simulink model "ELS_Testbench"  (R2021a)
settings: Solver=VariableStepAuto  StartTime=0.0  StopTime=10  FixedStep=Tsample  MaxStep=100e-4  RelTol=1e-3
values from neighbouring files (symbols this model uses):
  EncMaxSteps = 16777216    [ELS_Konstanten.m]
  EncOrTime = EncMaxSteps /(4096 * (RPM/60))    (= 144.564705882)    [ELS_Konstanten.m]
  TSampleRTM = 0.1e-3    (= 0.0001)    [ELS_Konstanten.m]
  TSampleStepper = 5e-6    (= 5e-06)    [ELS_Konstanten.m]
undefined symbols (not defined in the file or in its folder): sigbuilder_block
libraries: fl_lib x12, nesl_utility x5, simulink x2, ee_lib x2
settings Model: PacingRate=0.001800  OrderedModelArguments=off  Creator=lu  LastModifiedBy=lu
settings SolverCC: AlgebraicLoopSolver=TrustRegion  AutoInsertRateTranBlk=on
settings DebuggingCC: SFMachineParentedDataDiag=warning

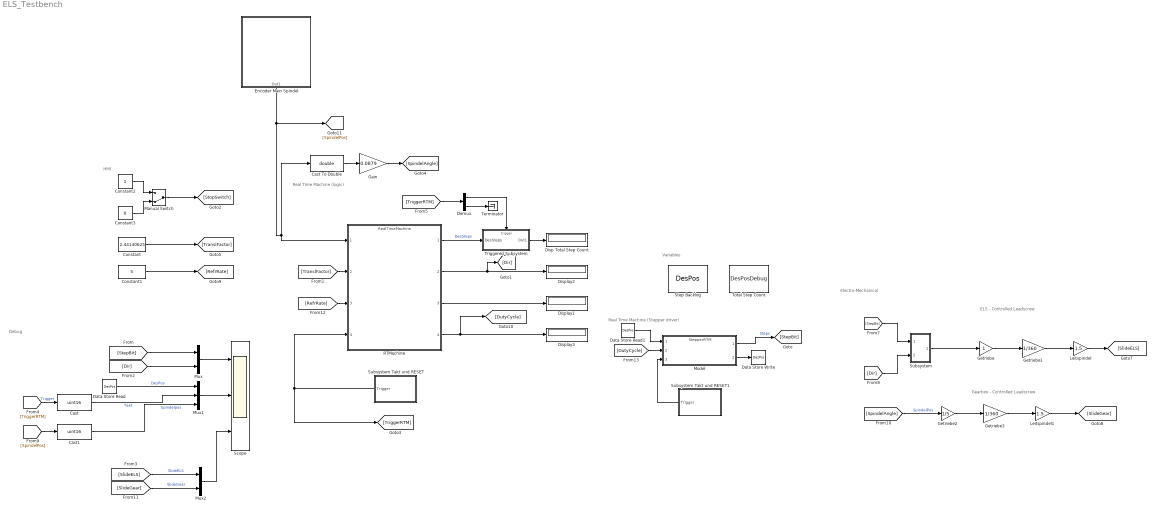
== system ELS_Testbench ==
  note: ELS - Controlled Leadscrew
  note: Electro-Mechanical
  note: Debug
  note: HMI
  note: Real Time Machine (Stepper driver)
  note: Real Time Machine (logic)
  note: Variables
  note: Gearbox - Controlled Leadscrew
  Cast : DataTypeConversion  OutDataTypeStr=uint16
  Cast To Double : DataTypeConversion  OutDataTypeStr=double
  Cast1 : DataTypeConversion  OutDataTypeStr=uint16
  Constant : Constant  Value=2.44140625  OutDataTypeStr=double
  Constant1 : Constant  Value=5  OutDataTypeStr=uint16
  Constant2 : Constant  OutDataTypeStr=boolean
  Constant3 : Constant  Value=0  OutDataTypeStr=boolean
  Data Store Read : DataStoreRead  DataStoreName=DesPos  IndexOptions=Index vector (dialog)  Indices=1  OutputSizes=1
  Data Store Read1 : DataStoreRead  DataStoreName=DesPos  IndexOptions=Index vector (dialog)  Indices=1  OutputSizes=1
  Data Store Write : DataStoreWrite  DataStoreName=DesPos  IndexOptions=Index vector (dialog)  Indices=1  OutputSizes=1
  Demux : Demux  Outputs=2
  Disp Total Step Count : Display
  Display1 : Display
  Display2 : Display
  Display3 : Display
  Encoder Main Spindel : Subsystem
  Gain : Gain  Gain=0.0879
  Getriebe : Gain
  Getriebe1 : Gain  Gain=1/360
  Getriebe2 : Gain  Gain=1/5
  Getriebe3 : Gain  Gain=1/360
  Leitspindel : Gain  Gain=1.5
  Leitspindel1 : Gain  Gain=1.5
  Manual Switch : ManualSwitch  CurrentSetting=0
  Model : ModelReference  ModelNameDialog=StepperRTM.slx  SimulationMode=Normal  ModelReferenceVersion=2.134
  Mux : Mux  Inputs=2
  Mux1 : Mux  Inputs=3
  Mux2 : Mux  Inputs=2
  RTMachine : ModelReference  ModelNameDialog=RealTimeMachine.slx  SimulationMode=Normal  ModelReferenceVersion=2.233
  Scope : Scope  NumInputPorts=3
  Step Backlog : DataStoreMemory  DataStoreName=DesPos  ReadBeforeWriteMsg=warning  WriteAfterWriteMsg=warning  WriteAfterReadMsg=warning  ShowAdditionalParam=off
  Subsystem : Subsystem
  Subsystem Takt und RESET : Subsystem
  Subsystem Takt und RESET1 : Subsystem
  Terminator : Terminator
  Total Step Count : DataStoreMemory  DataStoreName=DesPosDebug  ReadBeforeWriteMsg=warning  WriteAfterWriteMsg=warning  WriteAfterReadMsg=warning  ShowAdditionalParam=off
  Triggered Subsystem : Subsystem  TreatAsAtomicUnit=on
  wires:
  Constant3/1 -> Manual Switch/2
  Constant2/1 -> Manual Switch/1
  Subsystem Takt und RESET/1(Trigger) -> RTMachine/4, [TriggerRTM]
  Model/1 -> [StepBit]  "Steps"
  [StepBit] -> Mux/1
  Mux/1 -> Scope/1
  Subsystem Takt und RESET1/1(Trigger) -> Model/3
  [Dir] -> Mux/2
  RTMachine/1 -> Triggered Subsystem/1(DesSteps)  "DesSteps"
  [TriggerRTM] -> Demux/1
  Demux/1 -> Triggered Subsystem/Trigger
  Demux/2 -> Terminator/1
  Triggered Subsystem/1(Out1) -> Disp Total Step Count/1
  Encoder Main Spindel/1(Out1) -> [SpindelPos], Cast To Double/1, RTMachine/1
  [TranslFactor] -> RTMachine/2
  Manual Switch/1 -> [StopSwitch]
  Constant/1 -> [TranslFactor]
  [StepBit] -> Subsystem/1(In1)
  [Dir] -> Subsystem/2(In2)
  Subsystem/1(theta) -> Getriebe/1
  Gain/1 -> [SpindelAngle]
  Data Store Read/1 -> Mux1/1  "DesPos"
  Mux1/1 -> Scope/2
  Cast To Double/1 -> Gain/1
  Getriebe/1 -> Getriebe1/1
  Getriebe1/1 -> Leitspindel/1
  Mux2/1 -> Scope/3
  Leitspindel/1 -> [SlideELS]
  [SlideELS] -> Mux2/1  "SlideELS"
  Getriebe2/1 -> Getriebe3/1
  Getriebe3/1 -> Leitspindel1/1
  [SpindelAngle] -> Getriebe2/1  "SpindelPos"
  Leitspindel1/1 -> [SlideGear]
  [SlideGear] -> Mux2/2  "SlideGear"
  Constant1/1 -> [RefrRate]
  [DutyCycle] -> Model/2
  Model/2 -> Data Store Write/1
  Data Store Read1/1 -> Model/1
  [TriggerRTM] -> Cast/1  "Trigger"
  Cast/1 -> Mux1/2  "Takt"
  Cast1/1 -> Mux1/3  "Spindelpos"
  [SpindelPos] -> Cast1/1
  RTMachine/4 -> Display3/1, [DutyCycle]
  [RefrRate] -> RTMachine/3
  RTMachine/2 -> [Dir], Display2/1
  RTMachine/3 -> Display1/1

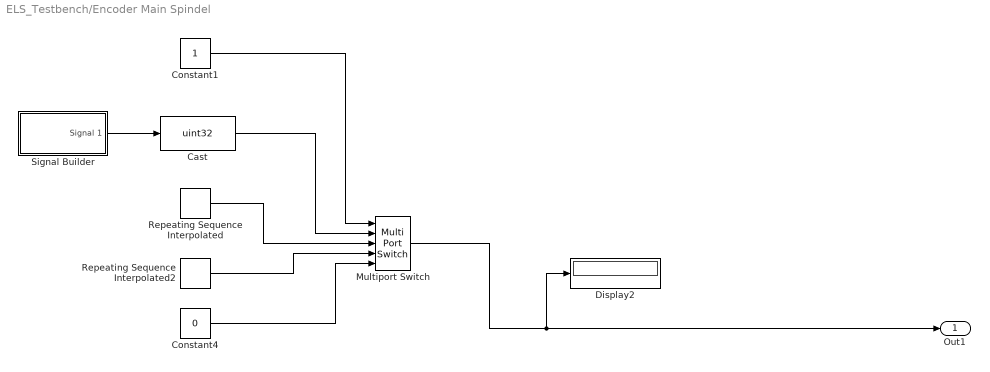
== system ELS_Testbench/Encoder Main Spindel ==
  Cast : DataTypeConversion  OutDataTypeStr=uint32
  Constant1 : Constant
  Constant4 : Constant  Value=0  OutDataTypeStr=uint32
  Display2 : Display
  Multiport Switch : MultiPortSwitch  Inputs=4
  Repeating Sequence Interpolated : simulink/Sources/Repeating Sequence Interpolated  OutValues=[0 EncMaxSteps/2 EncMaxSteps].'  TimeValues=[0 EncOrTime/2 EncOrTime].'  LookUpMeth=Interpolation-Use End Values  tsamp=TSampleRTM  OutMin=[]  OutMax=[]  OutDataTypeStr=uint32  OutputDataTypeScalingMode=uint32  OutDataType=fixdt(0,8)  OutScaling=2^-10
  Repeating Sequence Interpolated2 : simulink/Sources/Repeating Sequence Interpolated  OutValues=[EncMaxSteps EncMaxSteps/2 0].'  TimeValues=[0 EncOrTime/2 EncOrTime].'  LookUpMeth=Interpolation-Use End Values  tsamp=TSampleRTM  OutMin=[]  OutMax=[]  OutDataTypeStr=uint32  OutputDataTypeScalingMode=uint32  OutDataType=fixdt(0,8)  OutScaling=2^-10
  Signal Builder : Subsystem  Tag=STV Subsys  LoadFcn=sigbuilder_block('load');  StartFcn=sigbuilder_block('start');  StopFcn=sigbuilder_block('stop');  ClipboardFcn=sigbuilder_block('clipboard');  mask(Sigbuilder block){tuvar=[0:10]}
      mask help: Simulink:masks:SigbuilderBlock_MD
      mask init:
      | if ~strcmp(get_param(bdroot(gcbh),'SimulationStatus'),'stopped') tuvar = sigbuilder_block('maskInit'); end
      settings: CopyFcn=sigbuilder_block('copy');  DeleteFcn=sigbuilder_block('delete');  ModelCloseFcn=sigbuilder_block('modelClose');  PreSaveFcn=sigbuilder_block('preSave');  PauseFcn=sigbuilder_block('pause');  ContinueFcn=sigbuilder_block('continue');  NameChangeFcn=sigbuilder_block('namechange');  OpenFcn=sigbuilder_block('open',[437.6 199.2 550.4 400 ]);  CloseFcn=sigbuilder_block('close');
      mask Display: plot(0, 0, 100, 100,[2, 2, 32, 32, 2], [68, 8, 8, 68, 68],[32, 2], [38, 38], [32, 19, 2],[53, 60, 44], [32, 17, 17, 2],[16, 16, 31, 31]);txt = getActiveGroup(gcbh);text(2, 100, txt,'verticalAlignment', 'top');
  Out1 : Outport
  wires:
  Repeating Sequence Interpolated2/1 -> Multiport Switch/4
  Constant1/1 -> Multiport Switch/1
  Cast/1 -> Multiport Switch/2
  Constant4/1 -> Multiport Switch/5
  Multiport Switch/1 -> Out1/1, Display2/1
  Repeating Sequence Interpolated/1 -> Multiport Switch/3
  Signal Builder/1(Signal 1) -> Cast/1

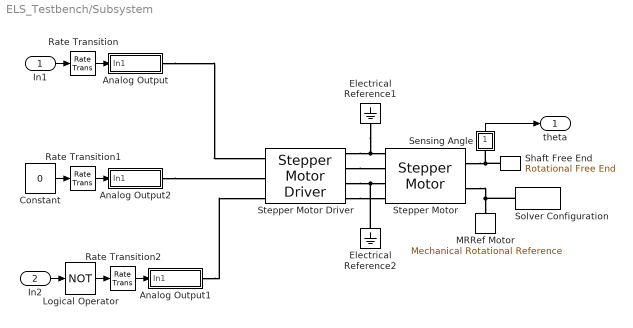
== system ELS_Testbench/Subsystem ==
  In1 : Inport
  In2 : Inport  Port=2
  Analog Output : Subsystem
  Analog Output1 : Subsystem
  Analog Output2 : Subsystem
  Constant : Constant  Value=0
  Electrical Reference1 : fl_lib/Electrical/Electrical Elements/Electrical Reference
  Electrical Reference2 : fl_lib/Electrical/Electrical Elements/Electrical Reference
  Logical Operator : Logic  Operator=NOT  AllPortsSameDT=off  OutDataTypeStr=boolean
  MRRef Motor : fl_lib/Mechanical/Rotational Elements/Mechanical Rotational Reference
  Rate Transition : RateTransition  Deterministic=off
  Rate Transition1 : RateTransition  Deterministic=off
  Rate Transition2 : RateTransition  Deterministic=off
  Sensing Angle : Subsystem
      mask Display: disp('a')
  Shaft Free End : fl_lib/Mechanical/Rotational Elements/Rotational Free End  w_specify=off  w_priority=None  w=0 rad/s  w_nominal_specify=off  w_nominal_unit=rad/s  w_nominal_value=1
      settings: SourceProductBaseCode=SS
  Solver Configuration : nesl_utility/Solver Configuration  PhysicalDomain=network_engine_domain  SubClassName=solver  LeftPortType=input  RightPortType=generic  Tones=[]  Harmonics=[]  SimulateNoise=off  Profile=off  UseLocalSampling=off  EnableSwitchedLinearOptims=on  FrequencyDomain=off  UseCCode=off  RelTol=0.001  AbsTol=1e-06  MinStep=1e-09  ToWorkspace=off  RevertToSquareIcSolve=off  NumHomotopyIterations=100  PhasorMode=off  PhasorModeNumHarmonics=1  DoDC=off  ResidualTolerance=1e-9  UseLocalSolver=off  LocalSolverChoice=NE_BACKWARD_EULER_ADVANCER  LocalSolverSampleTime=.001  DoFixedCost=off  MaxNonlinIter=3  MaxModeIter=2  ComputeImpulses=off  ImpulseIterations=2  LinearAlgebra=auto  EquationFormulation=NE_TIME_EF  DelaysMemoryBudget=1024  AutomaticFiltering=on  FilteringTimeConstant=3e-6  PartitionStorageMethod=AS_NEEDED  PartitionMemoryBudget=1024  PartitionMethod=FAST
      settings: SourceProductBaseCode=PW,SS
  Stepper Motor : ee_lib/Electromechanical/Reluctance & Stepper/Stepper Motor  Tag={'toolbox/physmod/elec/library/m/ee_lib_parts';'Electromechanical/Reluctance_and_Stepper/Stepper_Motor/Minebea/x08PM_K139BSTDCN.xml'}  step_or_av=1  w_vec=[0 1000 3000] rpm  T_vec=[2 2 1] N*m  assert_if_slipping=0  J_total=0.0001 kg*m^2  max_step_rate=10 Hz  Ra=6.5 Ohm  La=3.2 mH  Km=51.63 mN*m/A  Td=2.5 mN*m  Rm=Inf Ohm  Step=0.18 deg  J=2.9e-07 kg*m^2  B=2.65e-05 N*m/(rad/s)  speed0=0 rpm  theta0=0 deg  alpha=[0.00393 0.00393] 1/K  Tmeas=25 degC  T_vec2=[1.7 1.7 0.85] N*m  Tmeas2=125 degC  half_stepping=0  thermal_masses=[100 100] J/K  initial_temperatures=[25 25] degC  rotor_thermal_mass=50 J/K  rotor_initial_temperature=25 degC  Rm_percent_rotor=90
      settings: AttributesFormatString=Minebea:08PM-K139BSTDCN  SourceProductBaseCode=PS  InternalSimscapePortConfiguration="{\"Bottom\":[],\"Left\":[{\"id\":\"pA\",\"label\":\"A+\",\"type\":\"foundation.electrical.electrical\"},{\"id\":\"nA\",\"label\":\"A-\",\"type\":\"foundation.electrical.electrical\"},{\"id\":\"pB\",\"label\":\"B+\",\"type\":\"foundation.electrical.electrical\"},{\"id\":\"nB\",\"label\":\"B-\",\"type\":\"foundation.electrical.electrical\"}],\"Right\":[{\"id\":\"R\",\"label\":\"R\",\"type\":\"foundation.mechanical.rotational.rotational\"},{\"id\":\"C\",\"label\":\"C\",\"type\":\"foundation.mechanical.rotational.rotational\"}],\"Top\":[]}"
  Stepper Motor Driver : ee_lib/Electromechanical/Reluctance & Stepper/Stepper Motor Driver  step_or_av=1  step_rate_per_volt=10 Hz/V  Venable=3 V  Vreverse=3 V  Vm=24 V  half_stepping=0
      settings: SourceProductBaseCode=PS  InternalSimscapePortConfiguration="{\"Bottom\":[],\"Left\":[{\"id\":\"ENA\",\"label\":\"ENA\",\"type\":\"foundation.electrical.electrical\"},{\"id\":\"REF\",\"label\":\"REF\",\"type\":\"foundation.electrical.electrical\"},{\"id\":\"REV\",\"label\":\"REV\",\"type\":\"foundation.electrical.electrical\"}],\"Right\":[{\"id\":\"pA\",\"label\":\"A+\",\"type\":\"foundation.electrical.electrical\"},{\"id\":\"nA\",\"label\":\"A-\",\"type\":\"foundation.electrical.electrical\"},{\"id\":\"pB\",\"label\":\"B+\",\"type\":\"foundation.electrical.electrical\"},{\"id\":\"nB\",\"label\":\"B-\",\"type\":\"foundation.electrical.electrical\"}],\"Top\":[]}"
  theta : Outport
  wires:
  Sensing Angle/1(theta) -> theta/1
  In1/1 -> Rate Transition/1
  Rate Transition/1 -> Analog Output/1(In1)
  Constant/1 -> Rate Transition1/1
  Rate Transition1/1 -> Analog Output2/1(In1)
  Rate Transition2/1 -> Analog Output1/1(In1)
  In2/1 -> Logical Operator/1
  Logical Operator/1 -> Rate Transition2/1
  connections:
  Analog Output1/RConn1 -- Stepper Motor Driver/LConn3
  MRRef Motor/LConn1 -- Stepper Motor/RConn2 -- Solver Configuration/RConn1
  Analog Output/RConn1 -- Stepper Motor Driver/LConn1
  Stepper Motor Driver/RConn4 -- Stepper Motor/LConn4
  Stepper Motor Driver/RConn3 -- Electrical Reference2/LConn1 -- Stepper Motor/LConn3
  Stepper Motor Driver/RConn2 -- Stepper Motor/LConn2
  Analog Output2/RConn1 -- Stepper Motor Driver/LConn2
  Sensing Angle/LConn1 -- Stepper Motor/RConn1 -- Shaft Free End/LConn1
  Stepper Motor Driver/RConn1 -- Electrical Reference1/LConn1 -- Stepper Motor/LConn1

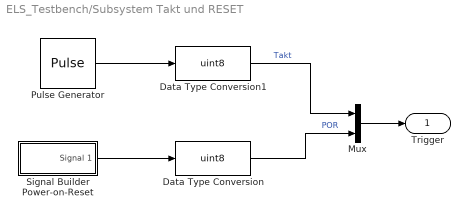
== system ELS_Testbench/Subsystem Takt und RESET ==
  Data Type Conversion : DataTypeConversion  OutDataTypeStr=uint8
  Data Type Conversion1 : DataTypeConversion  OutDataTypeStr=uint8
  Mux : Mux  Inputs=2
  Pulse Generator : DiscretePulseGenerator  SampleTime=TSampleRTM
  Signal Builder Power-on-Reset : Subsystem  Tag=STV Subsys  LoadFcn=sigbuilder_block('load');  StartFcn=sigbuilder_block('start');  StopFcn=sigbuilder_block('stop');  ClipboardFcn=sigbuilder_block('clipboard');  mask(Sigbuilder block){tuvar=[0:10]}
      mask help: Create and generate interchangeable groups of signals whose waveforms are piecewise linear.
      mask init:
      | if ~strcmp(get_param(bdroot(gcbh),'SimulationStatus'),'stopped') tuvar = sigbuilder_block('maskInit'); end
      settings: CopyFcn=sigbuilder_block('copy');  DeleteFcn=sigbuilder_block('delete');  ModelCloseFcn=sigbuilder_block('modelClose');  PreSaveFcn=sigbuilder_block('preSave');  PauseFcn=sigbuilder_block('pause')  ContinueFcn=sigbuilder_block('continue')  NameChangeFcn=sigbuilder_block('namechange');  OpenFcn=sigbuilder_block('open',[437.25 199.5 550.5 399.75 ]);  CloseFcn=sigbuilder_block('close');
      mask Display: plot(0, 0, 100, 100,[2, 2, 32, 32, 2], [68, 8, 8, 68, 68],[32, 2], [38, 38], [32, 19, 2],[53, 60, 44], [32, 17, 17, 2],[16, 16, 31, 31]);txt = getActiveGroup(gcbh);text(2, 100, txt,'verticalAlignment', 'top');
  Trigger : Outport  OutDataTypeStr=uint8  VectorParamsAs1DForOutWhenUnconnected=off
  wires:
  Signal Builder Power-on-Reset/1(Signal 1) -> Data Type Conversion/1
  Data Type Conversion/1 -> Mux/2  "POR"
  Mux/1 -> Trigger/1
  Pulse Generator/1 -> Data Type Conversion1/1
  Data Type Conversion1/1 -> Mux/1  "Takt"

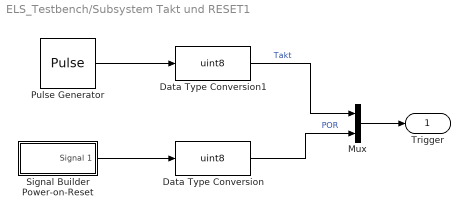
== system ELS_Testbench/Subsystem Takt und RESET1 ==
  Data Type Conversion : DataTypeConversion  OutDataTypeStr=uint8
  Data Type Conversion1 : DataTypeConversion  OutDataTypeStr=uint8
  Mux : Mux  Inputs=2
  Pulse Generator : DiscretePulseGenerator  SampleTime=TSampleStepper
  Signal Builder Power-on-Reset : Subsystem  Tag=STV Subsys  LoadFcn=sigbuilder_block('load');  StartFcn=sigbuilder_block('start');  StopFcn=sigbuilder_block('stop');  ClipboardFcn=sigbuilder_block('clipboard');  mask(Sigbuilder block){tuvar=[0:10]}
      mask help: Create and generate interchangeable groups of signals whose waveforms are piecewise linear.
      mask init:
      | if ~strcmp(get_param(bdroot(gcbh),'SimulationStatus'),'stopped') tuvar = sigbuilder_block('maskInit'); end
      settings: CopyFcn=sigbuilder_block('copy');  DeleteFcn=sigbuilder_block('delete');  ModelCloseFcn=sigbuilder_block('modelClose');  PreSaveFcn=sigbuilder_block('preSave');  PauseFcn=sigbuilder_block('pause')  ContinueFcn=sigbuilder_block('continue')  NameChangeFcn=sigbuilder_block('namechange');  OpenFcn=sigbuilder_block('open',[437.25 199.5 550.5 399.75 ]);  CloseFcn=sigbuilder_block('close');
      mask Display: plot(0, 0, 100, 100,[2, 2, 32, 32, 2], [68, 8, 8, 68, 68],[32, 2], [38, 38], [32, 19, 2],[53, 60, 44], [32, 17, 17, 2],[16, 16, 31, 31]);txt = getActiveGroup(gcbh);text(2, 100, txt,'verticalAlignment', 'top');
  Trigger : Outport  OutDataTypeStr=uint8  VectorParamsAs1DForOutWhenUnconnected=off
  wires:
  Signal Builder Power-on-Reset/1(Signal 1) -> Data Type Conversion/1
  Data Type Conversion/1 -> Mux/2  "POR"
  Mux/1 -> Trigger/1
  Pulse Generator/1 -> Data Type Conversion1/1
  Data Type Conversion1/1 -> Mux/1  "Takt"

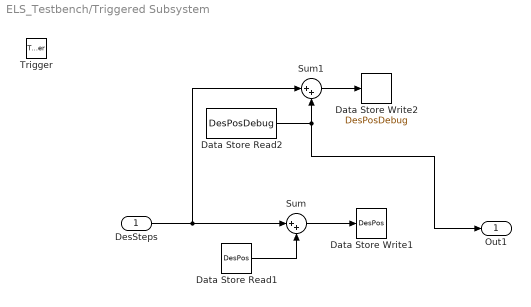
== system ELS_Testbench/Triggered Subsystem ==
  DesSteps : Inport
  Trigger : TriggerPort  TriggerType=either  VariantControl=(inherit)
  Data Store Read1 : DataStoreRead  DataStoreName=DesPos  IndexOptions=Index vector (dialog)  Indices=1  OutputSizes=1
  Data Store Read2 : DataStoreRead  DataStoreName=DesPosDebug  IndexOptions=Index vector (dialog)  Indices=1  OutputSizes=1
  Data Store Write1 : DataStoreWrite  DataStoreName=DesPos  IndexOptions=Index vector (dialog)  Indices=1  OutputSizes=1
  Data Store Write2 : DataStoreWrite  DataStoreName=DesPosDebug  IndexOptions=Index vector (dialog)  Indices=1  OutputSizes=1
  Sum : Sum  Inputs=|++
  Sum1 : Sum  Inputs=|++
  Out1 : Outport
  wires:
  Sum/1 -> Data Store Write1/1
  Data Store Read1/1 -> Sum/2
  DesSteps/1 -> Sum1/1, Sum/1
  Sum1/1 -> Data Store Write2/1
  Data Store Read2/1 -> Out1/1, Sum1/2

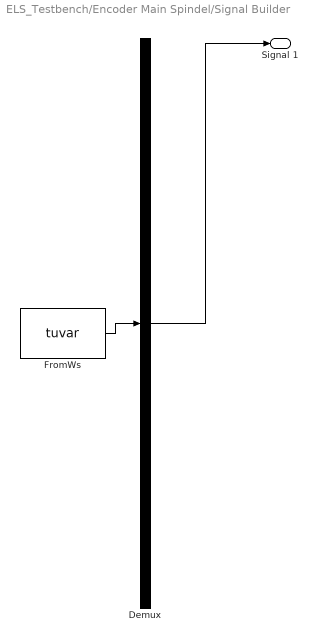
== system ELS_Testbench/Encoder Main Spindel/Signal Builder ==
  Demux : Demux  Tag=STV Demux  Outputs=1
      settings: DisplayOption=none
  FromWs : FromWorkspace  Tag=STV FromWs  VariableName=tuvar
      SigBuilderData=|
      | common.afterFinalStr = 'Extrapolate'
      | common.sampleTime = 0
      | dataSet.timeRange = [0 10]
      | dataSet.name = 'Group 1'
      | sbobj.Groups.Name = 'Group 1'
      | sbobj.Groups.Signals.Name = 'Signal 1'
      | sbobj.Groups.Signals.XData = [0 1 2 2.5 3 10]
      | sbobj.Groups.Signals.YData = [0 0 4096 4096 1000 0]
  Signal 1 : Outport  Tag=STV Outport
  wires:
  Demux/1 -> Signal 1/1
  FromWs/1 -> Demux/1

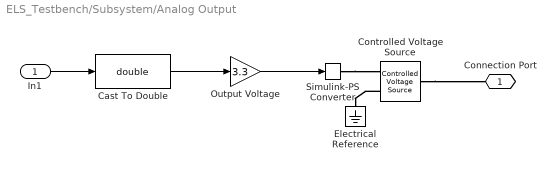
== system ELS_Testbench/Subsystem/Analog Output ==
  In1 : Inport
  Cast To Double : DataTypeConversion  OutDataTypeStr=double
  Controlled Voltage Source : fl_lib/Electrical/Electrical Sources/Controlled Voltage Source
  Electrical Reference : fl_lib/Electrical/Electrical Elements/Electrical Reference
  Output Voltage : Gain  Gain=3.3
  Simulink-PS Converter : nesl_utility/Simulink-PS Converter  PhysicalDomain=network_engine_domain  SubClassName=ps_input  LeftPortType=input  RightPortType=output  PseudoPeriodic=off  Frequencies=[]  NoiseDistribution=none  NoiseParameters=[]  Unit=1  AffineConversion=off  FilteringAndDerivatives=provide  SimscapeFilterOrder=1  InputFilterTimeConstant=0.001  UdotUserProvided=0
      settings: SourceProductBaseCode=PW,SS
  Connection Port : PMIOPort  Side=Right
  wires:
  In1/1 -> Cast To Double/1
  Output Voltage/1 -> Simulink-PS Converter/1
  Cast To Double/1 -> Output Voltage/1
  connections:
  Simulink-PS Converter/RConn1 -- Controlled Voltage Source/RConn1
  Controlled Voltage Source/LConn1 -- Connection Port/RConn1
  Controlled Voltage Source/RConn2 -- Electrical Reference/LConn1

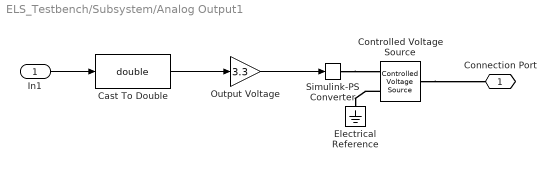
== system ELS_Testbench/Subsystem/Analog Output1 ==
  In1 : Inport
  Cast To Double : DataTypeConversion  OutDataTypeStr=double
  Controlled Voltage Source : fl_lib/Electrical/Electrical Sources/Controlled Voltage Source
  Electrical Reference : fl_lib/Electrical/Electrical Elements/Electrical Reference
  Output Voltage : Gain  Gain=3.3
  Simulink-PS Converter : nesl_utility/Simulink-PS Converter  PhysicalDomain=network_engine_domain  SubClassName=ps_input  LeftPortType=input  RightPortType=output  PseudoPeriodic=off  Frequencies=[]  NoiseDistribution=none  NoiseParameters=[]  Unit=1  AffineConversion=off  FilteringAndDerivatives=provide  SimscapeFilterOrder=1  InputFilterTimeConstant=0.001  UdotUserProvided=0
      settings: SourceProductBaseCode=PW,SS
  Connection Port : PMIOPort  Side=Right
  wires:
  Output Voltage/1 -> Simulink-PS Converter/1
  In1/1 -> Cast To Double/1
  Cast To Double/1 -> Output Voltage/1
  connections:
  Controlled Voltage Source/LConn1 -- Connection Port/RConn1
  Controlled Voltage Source/RConn2 -- Electrical Reference/LConn1
  Simulink-PS Converter/RConn1 -- Controlled Voltage Source/RConn1

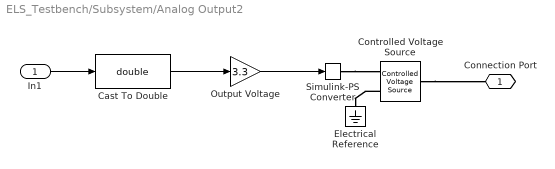
== system ELS_Testbench/Subsystem/Analog Output2 ==
  In1 : Inport
  Cast To Double : DataTypeConversion  OutDataTypeStr=double
  Controlled Voltage Source : fl_lib/Electrical/Electrical Sources/Controlled Voltage Source
  Electrical Reference : fl_lib/Electrical/Electrical Elements/Electrical Reference
  Output Voltage : Gain  Gain=3.3
  Simulink-PS Converter : nesl_utility/Simulink-PS Converter  PhysicalDomain=network_engine_domain  SubClassName=ps_input  LeftPortType=input  RightPortType=output  PseudoPeriodic=off  Frequencies=[]  NoiseDistribution=none  NoiseParameters=[]  Unit=1  AffineConversion=off  FilteringAndDerivatives=provide  SimscapeFilterOrder=1  InputFilterTimeConstant=0.001  UdotUserProvided=0
      settings: SourceProductBaseCode=PW,SS
  Connection Port : PMIOPort  Side=Right
  wires:
  In1/1 -> Cast To Double/1
  Output Voltage/1 -> Simulink-PS Converter/1
  Cast To Double/1 -> Output Voltage/1
  connections:
  Simulink-PS Converter/RConn1 -- Controlled Voltage Source/RConn1
  Controlled Voltage Source/LConn1 -- Connection Port/RConn1
  Controlled Voltage Source/RConn2 -- Electrical Reference/LConn1

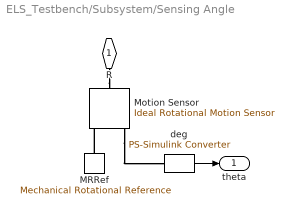
== system ELS_Testbench/Subsystem/Sensing Angle ==
  MRRef : fl_lib/Mechanical/Rotational Elements/Mechanical Rotational Reference
  Motion Sensor : fl_lib/Mechanical/Mechanical Sensors/Ideal Rotational Motion Sensor  wrap_angle=simscape.enum.onoff.off  offset=0 deg
  deg : nesl_utility/PS-Simulink Converter  PhysicalDomain=network_engine_domain  SubClassName=ps_output  LeftPortType=input  RightPortType=output  PseudoPeriodic=off  Frequencies=[]  Unit=deg  AffineConversion=off
      settings: SourceProductBaseCode=PW,SS
  R : PMIOPort  Side=Left
  theta : Outport  VectorParamsAs1DForOutWhenUnconnected=off
  wires:
  deg/1 -> theta/1
  connections:
  R/RConn1 -- Motion Sensor/LConn1
  Motion Sensor/RConn3 -- deg/LConn1
  MRRef/LConn1 -- Motion Sensor/RConn1

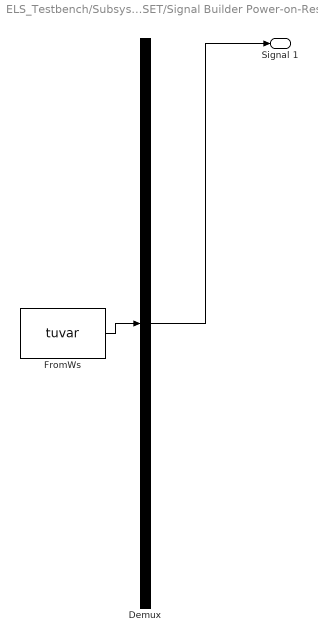
== system ELS_Testbench/Subsystem Takt und RESET/Signal Builder Power-on-Reset ==
  Demux : Demux  Tag=STV Demux  Outputs=1
      settings: DisplayOption=none
  FromWs : FromWorkspace  Tag=STV FromWs  VariableName=tuvar
      SigBuilderData=|
      | common.afterFinalStr = 'Extrapolate'
      | common.sampleTime = 0
      | dataSet.timeRange = [0 10]
      | dataSet.name = 'Group 1'
      | sbobj.Groups.Name = 'Group 1'
      | sbobj.Groups.Signals.Name = 'Signal 1'
      | sbobj.Groups.Signals.XData = [0 1 1 10]
      | sbobj.Groups.Signals.YData = [0 0 1 1]
  Signal 1 : Outport  Tag=STV Outport  VectorParamsAs1DForOutWhenUnconnected=off
  wires:
  Demux/1 -> Signal 1/1
  FromWs/1 -> Demux/1

== system ELS_Testbench/Subsystem Takt und RESET1/Signal Builder Power-on-Reset ==
  Demux : Demux  Tag=STV Demux  Outputs=1
      settings: DisplayOption=none
  FromWs : FromWorkspace  Tag=STV FromWs  VariableName=tuvar
      SigBuilderData=|
      | common.afterFinalStr = 'Extrapolate'
      | common.sampleTime = 0
      | dataSet.timeRange = [0 10]
      | dataSet.name = 'Group 1'
      | sbobj.Groups.Name = 'Group 1'
      | sbobj.Groups.Signals.Name = 'Signal 1'
      | sbobj.Groups.Signals.XData = [0 1 1 10]
      | sbobj.Groups.Signals.YData = [0 0 1 1]
  Signal 1 : Outport  Tag=STV Outport  VectorParamsAs1DForOutWhenUnconnected=off
  wires:
  Demux/1 -> Signal 1/1
  FromWs/1 -> Demux/1
